simulink model "TJA1042_Loop_Example"  (R2024a)
settings: Solver=FixedStepAuto  StartTime=0.0  StopTime=10.0  RelTol=1e-3
PreLoadFcn:
  | % NXP_MBDT_S32K3 callback: DO NOT REMOVE
  | mbd_s32k3.common.nxp.model_callbacks.preLoadFcn();
PostLoadFcn:
  | % NXP_MBDT_S32K3 callback: DO NOT REMOVE
  | mbd_s32k3.common.nxp.model_callbacks.postLoadFcn();
InitFcn:
  | % NXP_MBDT_S32K3 callback: DO NOT REMOVE
  | mbd_s32k3.common.nxp.model_callbacks.initFcn();
undefined symbols (not defined in the file or in its folder): mbd_s32k3
libraries: mbd_s32k3_communication_library x7, mbd_s32k3_io_library x5, mbd_s32k3_isr_library x1
(part 5 of 5)

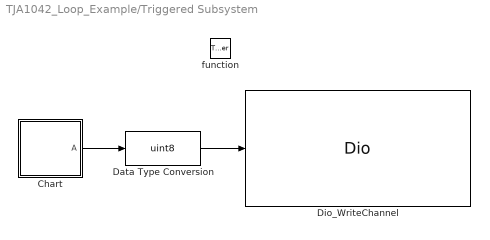
== system TJA1042_Loop_Example/Triggered Subsystem ==
  function : TriggerPort  TriggerType=function-call  VariantControl=Variant
  Chart : Stateflow chart  TreatAsAtomicUnit=on
  Data Type Conversion : DataTypeConversion  OutDataTypeStr=uint8  SaturateOnIntegerOverflow=off  RndMeth=Floor
  Dio_WriteChannel : mbd_s32k3_io_library/Dio  api_func=Dio_WriteChannel  channel=RGBLED0_BLUE  channel_group=No channel groups configured  port=PTA_H  gpioSim=on  text=<binary blob, 4382 chars, not shown>
      settings: SourceProductName=IO Blocks
  wires:
  Chart/1(" A") -> Data Type Conversion/1
  Data Type Conversion/1 -> Dio_WriteChannel/1

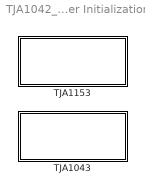
== system TJA1042_Loop_Example/Initialize Function/CAN Transceiver Initialization ==
  TJA1043 : Subsystem  VariantControl=TJA_SEL == 1043
  TJA1153 : Subsystem  VariantControl=(default)

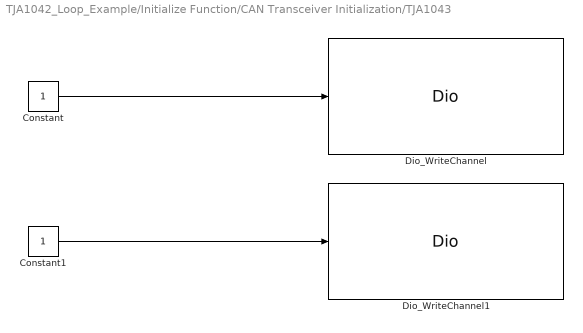
== system TJA1042_Loop_Example/Initialize Function/CAN Transceiver Initialization/TJA1043 ==
  Constant : Constant  OutDataTypeStr=uint8
  Constant1 : Constant  OutDataTypeStr=uint8
  Dio_WriteChannel : mbd_s32k3_io_library/Dio  api_func=Dio_WriteChannel  channel=CAN0_EN_NXP  channel_group=No channel groups configured  port=PTA_H  gpioSim=on  text=<binary blob, 4382 chars, not shown>
      settings: SourceProductName=IO Blocks
  Dio_WriteChannel1 : mbd_s32k3_io_library/Dio  api_func=Dio_WriteChannel  channel=CAN0_STB_NXP  channel_group=No channel groups configured  port=PTA_H  gpioSim=on  text=<binary blob, 4382 chars, not shown>
      settings: SourceProductName=IO Blocks
  wires:
  Constant/1 -> Dio_WriteChannel/1
  Constant1/1 -> Dio_WriteChannel1/1

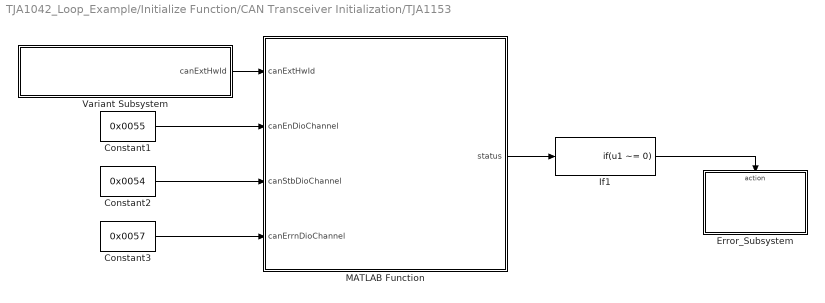
== system TJA1042_Loop_Example/Initialize Function/CAN Transceiver Initialization/TJA1153 ==
  Constant1 : Constant  Value=0x0055  OutDataTypeStr=uint16
  Constant2 : Constant  Value=0x0054  OutDataTypeStr=uint16
  Constant3 : Constant  Value=0x0057  OutDataTypeStr=uint16
  Error_Subsystem : Subsystem
  If1 : If  IfExpression=u1 ~= 0  ShowElse=off
  MATLAB Function : MATLAB Function  TreatAsAtomicUnit=on
  Variant Subsystem : Subsystem  Variant=on
  wires:
  MATLAB Function/1(status) -> If1/1
  If1/1 -> Error_Subsystem/Action
  Constant1/1 -> MATLAB Function/2(canEnDioChannel)
  Constant2/1 -> MATLAB Function/3(canStbDioChannel)
  Constant3/1 -> MATLAB Function/4(canErrnDioChannel)
  Variant Subsystem/1(canExtHwId) -> MATLAB Function/1(canExtHwId)

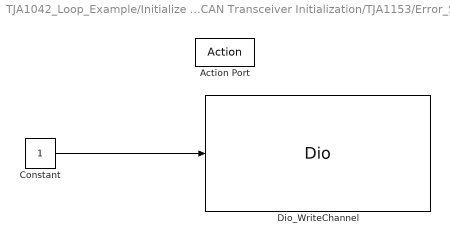
== system TJA1042_Loop_Example/Initialize Function/CAN Transceiver Initialization/TJA1153/Error_Subsystem ==
  Action Port : ActionPort
  Constant : Constant  OutDataTypeStr=Inherit: Inherit via back propagation
  Dio_WriteChannel : mbd_s32k3_io_library/Dio  api_func=Dio_WriteChannel  channel=RGBLED0_RED  channel_group=No channel groups configured  port=PTA_H  gpioSim=on  text=<binary blob, 4382 chars, not shown>
      settings: SourceProductName=IO Blocks
  wires:
  Constant/1 -> Dio_WriteChannel/1

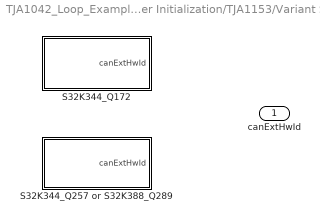
== system TJA1042_Loop_Example/Initialize Function/CAN Transceiver Initialization/TJA1153/Variant Subsystem ==
  S32K344_Q172 : Subsystem  VariantControl=strcmp(mbd_s32k3.common.nxp.utils.get_hardware_type, 'S32K344-Q172')
  S32K344_Q257 or S32K388_Q289 : Subsystem  VariantControl=(default)
  canExtHwId : Outport

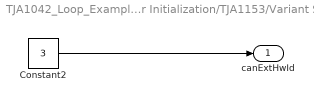
== system TJA1042_Loop_Example/Initialize Function/CAN Transceiver Initialization/TJA1153/Variant Subsystem/S32K344_Q172 ==
  Constant2 : Constant  Value=3  OutDataTypeStr=uint16
  canExtHwId : Outport
  wires:
  Constant2/1 -> canExtHwId/1

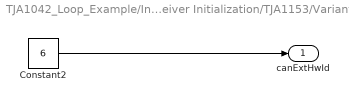
== system TJA1042_Loop_Example/Initialize Function/CAN Transceiver Initialization/TJA1153/Variant Subsystem/S32K344_Q257 or S32K388_Q289 ==
  Constant2 : Constant  Value=6  OutDataTypeStr=uint16
  canExtHwId : Outport
  wires:
  Constant2/1 -> canExtHwId/1

== stateflow chart TJA1042_Loop_Example/Triggered Subsystem/Chart ==
  state A
  state A1
  (default) -> A
  A -> A1
  A1 -> A
  data: A output boolean [0..1]

== matlab function TJA1042_Loop_Example/Initialize Function/CAN Transceiver Initialization/TJA1153/MATLAB Function ==
  data: status output; canExtHwId input; canEnDioChannel input; canStbDioChannel input; canErrnDioChannel input
function status = TJA1153_Init(canExtHwId, canEnDioChannel, canStbDioChannel, canErrnDioChannel)

	status = mbd_s32k3.common.nxp.can.TJA1153Transceiver.init(canExtHwId, canEnDioChannel, canStbDioChannel, canErrnDioChannel);

end
